simulink subsystem "ArduinoController2"  (R2020a)
settings: Solver=VariableStepAuto  StartTime=0.0  StopTime=10.0  RelTol=1e-3
model mask{dsys=mModel{nodeID,3}, C=C', Ts=Ts, vphi=vphi, gamm=gamm, delt=del, qT=qT, xiT=xiT, eta=eta, N=N}
  mask prompts: dsys "model"; vphi "varphi"; gamm "gamma"; delt "delta"
values from neighbouring files (symbols this model uses):
  C = single(Cs(nodeID,:))    [ParamSetup.m]
  eta = single(etas(nodeID))    [ParamSetup.m]
  gamm = single(gamms(nodeID))    [ParamSetup.m]
  N = uint8(10)    [ParamSetup.m]
  qT = single(qTs(nodeID))    [ParamSetup.m]
  Ts = 0.015    [ParamSetup.m]    (also in motorModel.mat = 0.002)
  vphi = single(vphis(nodeID))    [ParamSetup.m]
  xiT = single(xiTs(nodeID))    [ParamSetup.m]
libraries: simulink x1
settings Model: Creator=khoi  LastModifiedBy=khoi

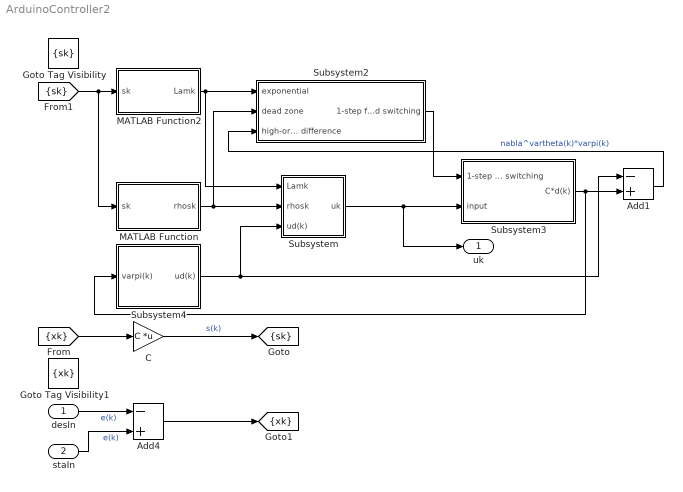
== system ArduinoController2 ==
  desIn : Inport
  staIn : Inport  Port=2
  Add1 : Sum  Inputs=-+
  Add4 : Sum  Inputs=-+
  C : Gain  Gain=C  Multiplication=Matrix(K*u) (u vector)
  Goto Tag Visibility : GotoTagVisibility  GotoTag=sk
  Goto Tag Visibility1 : GotoTagVisibility  GotoTag=xk
  MATLAB Function : MATLAB Function  TreatAsAtomicUnit=on  mask{eta=eta}
      mask prompts: eta "eta>0"
  MATLAB Function2 : MATLAB Function  TreatAsAtomicUnit=on  mask{del=delt, vphi=vphi, gam=round(gamm)}
      mask prompts: del "0<delta<1"; vphi "vphi>0"; gam "gamma>0 natrual number"
  Subsystem : Subsystem
  Subsystem2 : Subsystem
  Subsystem3 : Subsystem
  Subsystem4 : Subsystem
  uk : Outport
  tag scope: sk=scoped, xk=scoped
  wires:
  Subsystem3/1(C*d(k)) -> Add1/2, Subsystem4/1(varpi(k))
  Subsystem/1(uk) -> uk/1, Subsystem3/2(input)
  [sk] -> MATLAB Function2/1(sk), MATLAB Function/1(sk)
  Subsystem2/1(1-step forward switching) -> Subsystem3/1(1-step forward switching)
  MATLAB Function2/1(Lamk) -> Subsystem2/1(exponential), Subsystem/1(Lamk)
  Subsystem4/1(ud(k)) -> Subsystem/3(ud(k)), Add1/1
  desIn/1 -> Add4/1  "e(k)"
  Add1/1 -> Subsystem2/3(high-order difference)  "nabla^vartheta(k)*varpi(k)"
  [xk] -> C/1
  C/1 -> [sk]  "s(k)"
  MATLAB Function/1(rhosk) -> Subsystem/2(rhosk), Subsystem2/2(dead zone)
  staIn/1 -> Add4/2  "e(k)"
  Add4/1 -> [xk]

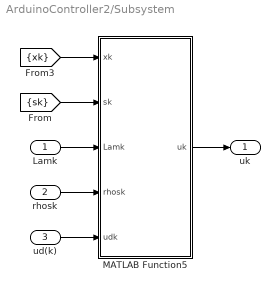
== system ArduinoController2/Subsystem ==
  Lamk : Inport
  rhosk : Inport  Port=2
  ud(k) : Inport  Port=3
  MATLAB Function5 : MATLAB Function  TreatAsAtomicUnit=on  mask{Phi=dsys.A, Gam=dsys.B, C=C, qT=qT, xiT=xiT}
  uk : Outport
  wires:
  [sk] -> MATLAB Function5/2(sk)
  rhosk/1 -> MATLAB Function5/4(rhosk)
  Lamk/1 -> MATLAB Function5/3(Lamk)
  MATLAB Function5/1(uk) -> uk/1
  ud(k)/1 -> MATLAB Function5/5(udk)
  [xk] -> MATLAB Function5/1(xk)

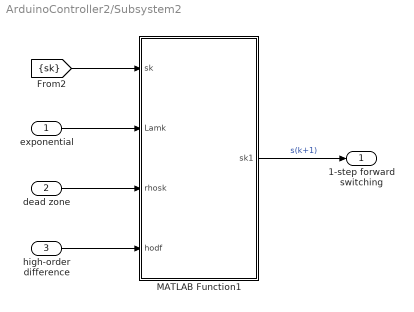
== system ArduinoController2/Subsystem2 ==
  exponential : Inport
  dead zone : Inport  Port=2
  high-order difference : Inport  Port=3
  MATLAB Function1 : MATLAB Function  TreatAsAtomicUnit=on  mask{xiT=xiT, qT=qT}
      mask prompts: xiT "xi > 0 (xiT>0)"; qT "q (0<1-qT<1)"
  1-step forward switching : Outport
  wires:
  exponential/1 -> MATLAB Function1/2(Lamk)
  dead zone/1 -> MATLAB Function1/3(rhosk)
  high-order difference/1 -> MATLAB Function1/4(hodf)
  MATLAB Function1/1(sk1) -> 1-step forward switching/1  "s(k+1)"
  [sk] -> MATLAB Function1/1(sk)

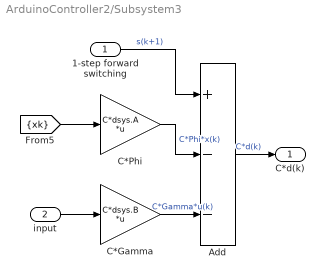
== system ArduinoController2/Subsystem3 ==
  1-step forward switching : Inport
  input : Inport  Port=2
  Add : Sum  Inputs=+--
  C*Gamma : Gain  Gain=C*dsys.B  Multiplication=Matrix(K*u)
  C*Phi : Gain  Gain=C*dsys.A  Multiplication=Matrix(K*u) (u vector)
  C*d(k) : Outport
  wires:
  1-step forward switching/1 -> Add/1  "s(k+1)"
  [xk] -> C*Phi/1
  Add/1 -> C*d(k)/1  "C*d(k)"
  input/1 -> C*Gamma/1
  C*Phi/1 -> Add/2  "C*Phi*x(k)"
  C*Gamma/1 -> Add/3  "C*Gamma*u(k)"

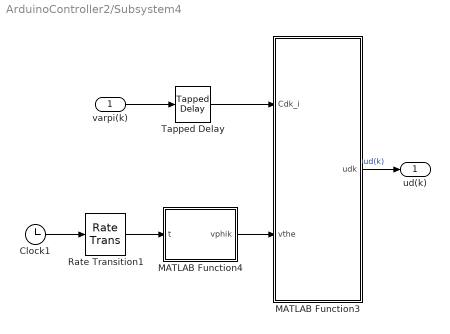
== system ArduinoController2/Subsystem4 ==
  varpi(k) : Inport
  Clock1 : Clock
  MATLAB Function3 : MATLAB Function  TreatAsAtomicUnit=on
  MATLAB Function4 : MATLAB Function  TreatAsAtomicUnit=on  mask{Ts=Ts, n=round(N)}
  Rate Transition1 : RateTransition  OutPortSampleTime=Ts
  Tapped Delay : simulink/Discrete/Tapped Delay  vinit=0.0  samptime=-1  NumDelays=round(N)  DelayOrder=Newest  includeCurrent=off
  ud(k) : Outport
  wires:
  MATLAB Function3/1(udk) -> ud(k)/1  "ud(k)"
  varpi(k)/1 -> Tapped Delay/1
  MATLAB Function4/1(vphik) -> MATLAB Function3/2(vthe)
  Rate Transition1/1 -> MATLAB Function4/1(t)
  Clock1/1 -> Rate Transition1/1
  Tapped Delay/1 -> MATLAB Function3/1(Cdk_i)

== matlab function ArduinoController2/MATLAB Function ==
  data: sk input; rhosk output; eta parameter
function rhosk = fDeadzone(sk,eta)
    if sk>eta
        rhosk=1;
    elseif abs(sk)<=eta
        rhosk=0;
    else % sk<-eta
        rhosk=-1;
    end

== matlab function ArduinoController2/MATLAB Function2 ==
  data: sk input; Lamk output; del parameter; vphi parameter; gam parameter
function Lamk = fLambda(sk,del,vphi,gam)
Lamk= del + (1-del)*exp(-vphi*abs(sk)^gam);

== matlab function ArduinoController2/Subsystem4/MATLAB Function4 ==
  data: t input; vphik output; Ts parameter; n parameter
function vphik = fVphi(t,Ts,n)
persistent k;
if isempty(k)
    k=0;
end
if rem(t,Ts)==0 && t~=0 && k<n
    k = k+1;
end
vphik = k;

== matlab function ArduinoController2/Subsystem2/MATLAB Function1 ==
  data: sk input; sk1 output; Lamk input; rhosk input; hodf input; xiT parameter; qT parameter
function sk1 = fFwrdSwit(sk,Lamk,rhosk,hodf,...
    xiT, qT)

sk1 = (1-qT)*Lamk*sk - xiT/Lamk*rhosk + hodf;

== matlab function ArduinoController2/Subsystem4/MATLAB Function3 ==
  data: Cdk_i input; vthe input; udk output
function udk = fDtbCompen(Cdk_i,vthe)
udk = 0;
for i=1:vthe
    udk = udk - (-1)^i*nchoosek(vthe,i)*Cdk_i(i);
end

== matlab function ArduinoController2/Subsystem/MATLAB Function5 ==
  data: xk input; uk output; sk input; Lamk input; rhosk input; udk input; Phi parameter; Gam parameter; C parameter; qT parameter; xiT parameter
function uk = fcn(xk,sk,Lamk,rhosk,udk,...
    Phi, Gam, C, qT, xiT)

uk = -(C*Gam)\(C*Phi*xk - (1-qT)*Lamk*sk + xiT/Lamk*rhosk + udk);
